simulink model "fortniteV2Sim"  (R2023b)
settings: Solver=FixedStepAuto  StartTime=0.0  StopTime=10.0  FixedStep=0.0001  RelTol=1e-3
values from neighbouring files (symbols this model uses):
  A = [0 0 0 0 1 0 0 0 ... (first row only)    [ME226_Problem6.m]
  B = [ ... (first row only)    [ME226_Problem6.m]
  C = [cs -cs ... (first row only)    [Final_Q3.m]    (also in ME226_Problem6.m = [1 0 0 0 0 0 0 0)
  D = zeros(8,2)    [ME226_Problem6.m]
settings Model: Creator=elija  LastModifiedBy=elija

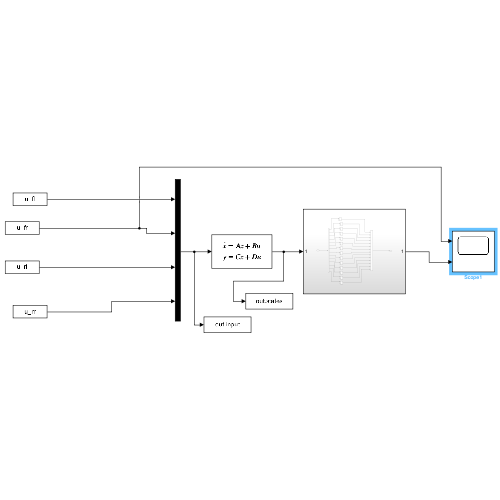
[thumbnail: Simulink's stored preview of the top-level diagram]
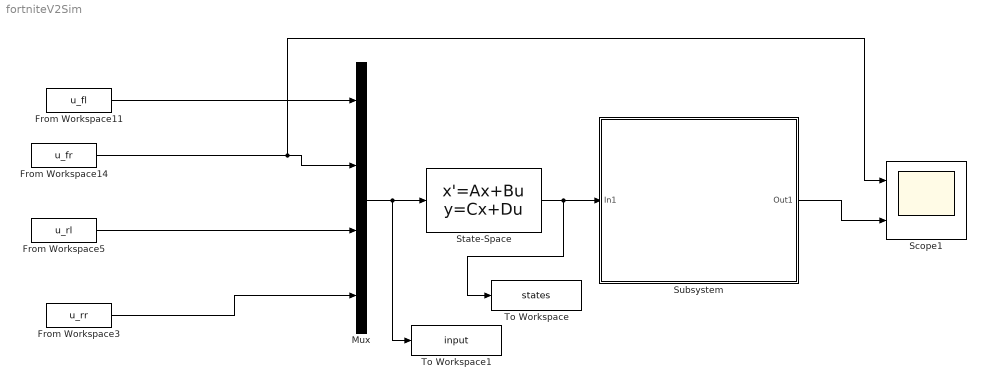
== system fortniteV2Sim ==
  From Workspace11 : FromWorkspace  VariableName=u_fl
  From Workspace14 : FromWorkspace  VariableName=u_fr
  From Workspace3 : FromWorkspace  VariableName=u_rr
  From Workspace5 : FromWorkspace  VariableName=u_rl
  Mux : Mux
  Scope1 : Scope  NumInputPorts=2
  State-Space : StateSpace  A=A  B=B  C=C  D=D  InitialCondition=0
  Subsystem : Subsystem
  To Workspace : ToWorkspace  VariableName=states  SaveFormat=Timeseries  SampleTime=-1
  To Workspace1 : ToWorkspace  VariableName=input  SaveFormat=Timeseries  SampleTime=-1
  wires:
  From Workspace3/1 -> Mux/4
  Mux/1 -> To Workspace1/1, State-Space/1
  State-Space/1 -> To Workspace/1, Subsystem/1(In1)
  Subsystem/1(Out1) -> Scope1/2
  From Workspace5/1 -> Mux/3
  From Workspace11/1 -> Mux/1
  From Workspace14/1 -> Scope1/1, Mux/2

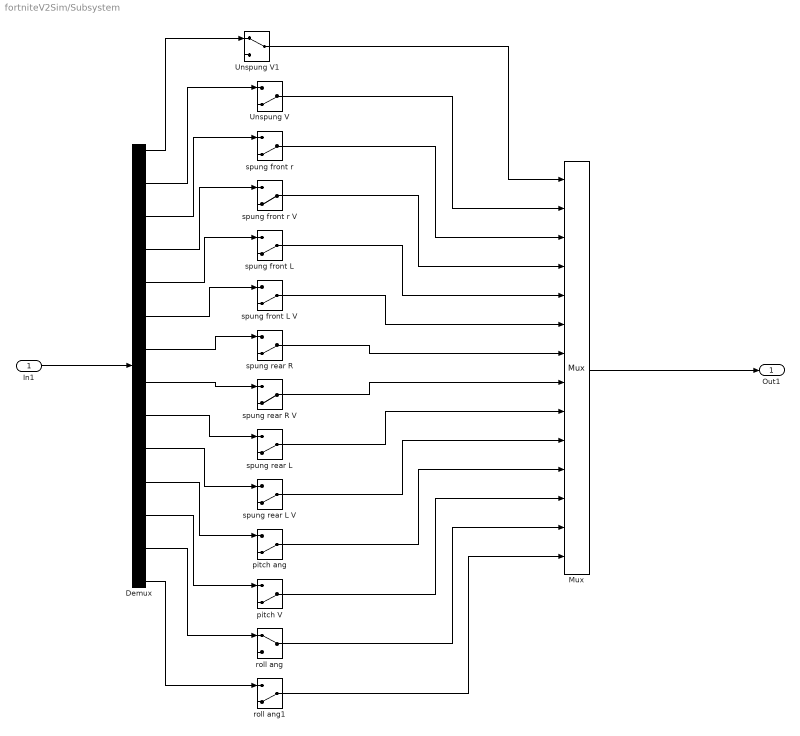
== system fortniteV2Sim/Subsystem ==
  In1 : Inport
  Demux : Demux  Outputs=14
  Mux : Mux  Inputs=14
  Unspung V : ManualSwitch  CurrentSetting=0
  Unspung V1 : ManualSwitch
  pitch V : ManualSwitch  CurrentSetting=0
  pitch ang : ManualSwitch  CurrentSetting=0
  roll ang : ManualSwitch
  roll ang1 : ManualSwitch  CurrentSetting=0
  spung front L : ManualSwitch  CurrentSetting=0
  spung front L V : ManualSwitch  CurrentSetting=0
  spung front r : ManualSwitch  CurrentSetting=0
  spung front r V : ManualSwitch  CurrentSetting=0
  spung rear L : ManualSwitch  CurrentSetting=0
  spung rear L V : ManualSwitch  CurrentSetting=0
  spung rear R : ManualSwitch  CurrentSetting=0
  spung rear R V : ManualSwitch  CurrentSetting=0
  Out1 : Outport
  wires:
  In1/1 -> Demux/1
  spung rear L/1 -> Mux/9
  spung rear R/1 -> Mux/7
  pitch ang/1 -> Mux/11
  Demux/12 -> pitch V/1
  Demux/6 -> spung front L V/1
  Demux/5 -> spung front L/1
  Demux/10 -> spung rear L V/1
  Demux/2 -> Unspung V/1
  Demux/9 -> spung rear L/1
  roll ang/1 -> Mux/13
  Demux/3 -> spung front r/1
  spung front L V/1 -> Mux/6
  spung front L/1 -> Mux/5
  Demux/4 -> spung front r V/1
  Demux/13 -> roll ang/1
  roll ang1/1 -> Mux/14
  Unspung V/1 -> Mux/2
  Demux/8 -> spung rear R V/1
  Demux/7 -> spung rear R/1
  Unspung V1/1 -> Mux/1
  pitch V/1 -> Mux/12
  spung front r/1 -> Mux/3
  spung rear L V/1 -> Mux/10
  spung front r V/1 -> Mux/4
  spung rear R V/1 -> Mux/8
  Demux/11 -> pitch ang/1
  Demux/1 -> Unspung V1/1
  Mux/1 -> Out1/1
  Demux/14 -> roll ang1/1
